simulink model "SecRwLtStLgrstInwdOtwdCtrl"  (R2018b)
settings: Solver=FixedStepDiscrete  StartTime=0.0  StopTime=10.0  FixedStep=0.01  RelTol=1e-3
undefined symbols (not defined in the file or in its folder): KeSMSuMdMotFinshdTm_Val, KeSMSuMdRetryTm1_Val, KeSMSuModeReqDurgTm_Val, KeSMSwSecRwLtStLgrstInwdOtwdEnTrigBitMask_Val
libraries: StCtrlLibBkRecln x1
settings Model: Creator=sn2xws  LastModifiedBy=sn55gm
settings Model: ModifiedHistory=|
  | 2024.10.14 V3.0.0 BitMask接口改为变量接口
  | 25.7.7 V3.13.0 Md61 Md62新增Retry口
  | 25.12.04 V3.14.0 MD10防夹后退出
settings DataIOCC: SaveFormat=StructureWithTime
settings OptimizationCC: DefaultParameterBehavior=Inlined  EnhancedBackFolding=on  PassReuseOutputArgsAs=Individual arguments  ZeroExternalMemoryAtStartup=off  ZeroInternalMemoryAtStartup=off  OptimizeBlockOrder=speed  DifferentSizesBufferReuse=on  OptimizationCustomize=off
settings DebuggingCC: ParameterTunabilityLossMsg=error
settings ModelReferenceCC: ModelReferenceNumInstancesAllowed=Single
settings SFSimCC: MATLABDynamicMemAlloc=off
settings RTWCC: SystemTargetFile=autosar.tlc  GenCodeOnly=on  TemplateMakefile=ert_default_tmf  Description=AUTOSAR  GenerateReport=on  IncludeHyperlinkInReport=on  LaunchReport=on  GenerateTraceInfo=on  GenerateTraceReport=on  GenerateTraceReportSl=on  GenerateTraceReportSf=on  GenerateTraceReportEml=on
settings CodeAppCC: ForceParamTrailComments=on  IgnoreCustomStorageClasses=off  OperatorAnnotations=on  SimulinkDataObjDesc=on  SFDataObjDesc=on  InsertBlockDesc=on
settings STFCustomTargetCC: TargetLangStandard=C99 (ISO)  MultiwordLength=256  ParMdlRefBuildCompliant=on  CompOptLevelCompliant=on  IncludeMdlTerminateFcn=off  CombineOutputUpdateFcns=on  SuppressErrorStatus=on  ERTCustomFileBanners=on  SupportNonFinite=off  SupportComplex=off  SupportContinuousTime=off  SupportNonInlinedSFcns=off  RemoveResetFunc=on  MATLABClassNameForMDSCustomization=Simulink.SoftwareTarget.ERTCustomization  AutosarCompliant=on  UseToolchainInfoCompliant=on  LookupTableObjectStructAxisOrder=2,1,3,4,...  LUTObjectStructOrderEvenSpacing=Size,Table,Breakpoints  SystemTargetFile=autosar.tlc
settings ERTTargetCC: TargetLangStandard=C99 (ISO)  ConcurrentExecutionCompliant=off  IncludeMdlTerminateFcn=off  SuppressErrorStatus=on  SupportNonFinite=off  SupportComplex=off  ModelStepFunctionPrototypeControlCompliant=off  CPPClassGenCompliant=off  AutosarCompliant=on  LookupTableObjectStructAxisOrder=2,1,3,4,...  LUTObjectStructOrderEvenSpacing=Size,Table,Breakpoints  InlinedParameterPlacement=NonHierarchical  ERTCustomFileTemplate=example_file_process.tlc  ERTFilePackagingFormat=Compact

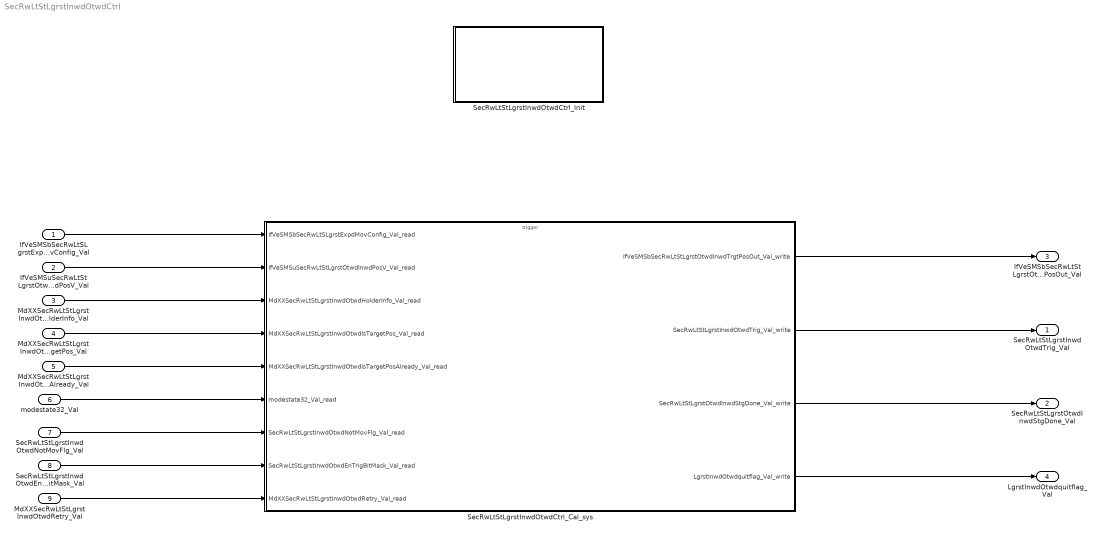
== system SecRwLtStLgrstInwdOtwdCtrl ==
  IfVeSMSbSecRwLtSLgrstExpdMovConfig_Val : Inport  OutDataTypeStr=boolean  PortDimensions=1
  IfVeSMSuSecRwLtStLgrstOtwdInwdPosV_Val : Inport  Port=2  OutDataTypeStr=boolean  PortDimensions=1
  MdXXSecRwLtStLgrstInwdOtwdHolderInfo_Val : Inport  Port=3  OutDataTypeStr=uint32  PortDimensions=1
  MdXXSecRwLtStLgrstInwdOtwdIsTargetPos_Val : Inport  Port=4  OutDataTypeStr=uint32  PortDimensions=1
  MdXXSecRwLtStLgrstInwdOtwdIsTargetPosAlready_Val : Inport  Port=5  OutDataTypeStr=uint32  PortDimensions=1
  modestate32_Val : Inport  Port=6  OutDataTypeStr=uint32  PortDimensions=1
  SecRwLtStLgrstInwdOtwdNotMovFlg_Val : Inport  Port=7  OutDataTypeStr=boolean  PortDimensions=1
  SecRwLtStLgrstInwdOtwdEnTrigBitMask_Val : Inport  Port=8  OutDataTypeStr=uint32  PortDimensions=1
  MdXXSecRwLtStLgrstInwdOtwdRetry_Val : Inport  Port=9  OutDataTypeStr=uint32  PortDimensions=1
  SecRwLtStLgrstInwdOtwdCtrl_Cal_sys : Subsystem
  SecRwLtStLgrstInwdOtwdCtrl_Init : Subsystem
  SecRwLtStLgrstInwdOtwdTrig_Val : Outport  OutDataTypeStr=boolean  PortDimensions=1
  SecRwLtStLgrstOtwdInwdStgDone_Val : Outport  Port=2  OutDataTypeStr=boolean  PortDimensions=1
  IfVeSMSbSecRwLtStLgrstOtwdInwdTrgtPosOut_Val : Outport  Port=3  OutDataTypeStr=boolean  PortDimensions=1
  LgrstInwdOtwdquitflag_Val : Outport  Port=4  OutDataTypeStr=boolean  PortDimensions=1
  wires:
  IfVeSMSbSecRwLtSLgrstExpdMovConfig_Val/1 -> SecRwLtStLgrstInwdOtwdCtrl_Cal_sys/1(IfVeSMSbSecRwLtSLgrstExpdMovConfig_Val_read)
  IfVeSMSuSecRwLtStLgrstOtwdInwdPosV_Val/1 -> SecRwLtStLgrstInwdOtwdCtrl_Cal_sys/2(IfVeSMSuSecRwLtStLgrstOtwdInwdPosV_Val_read)
  MdXXSecRwLtStLgrstInwdOtwdHolderInfo_Val/1 -> SecRwLtStLgrstInwdOtwdCtrl_Cal_sys/3(MdXXSecRwLtStLgrstInwdOtwdHolderInfo_Val_read)
  MdXXSecRwLtStLgrstInwdOtwdIsTargetPos_Val/1 -> SecRwLtStLgrstInwdOtwdCtrl_Cal_sys/4(MdXXSecRwLtStLgrstInwdOtwdIsTargetPos_Val_read)
  MdXXSecRwLtStLgrstInwdOtwdIsTargetPosAlready_Val/1 -> SecRwLtStLgrstInwdOtwdCtrl_Cal_sys/5(MdXXSecRwLtStLgrstInwdOtwdIsTargetPosAlready_Val_read)
  modestate32_Val/1 -> SecRwLtStLgrstInwdOtwdCtrl_Cal_sys/6(modestate32_Val_read)
  SecRwLtStLgrstInwdOtwdNotMovFlg_Val/1 -> SecRwLtStLgrstInwdOtwdCtrl_Cal_sys/7(SecRwLtStLgrstInwdOtwdNotMovFlg_Val_read)
  SecRwLtStLgrstInwdOtwdCtrl_Cal_sys/1(IfVeSMSbSecRwLtStLgrstOtwdInwdTrgtPosOut_Val_write) -> IfVeSMSbSecRwLtStLgrstOtwdInwdTrgtPosOut_Val/1
  SecRwLtStLgrstInwdOtwdCtrl_Cal_sys/2(SecRwLtStLgrstInwdOtwdTrig_Val_write) -> SecRwLtStLgrstInwdOtwdTrig_Val/1
  SecRwLtStLgrstInwdOtwdCtrl_Cal_sys/3(SecRwLtStLgrstOtwdInwdStgDone_Val_write) -> SecRwLtStLgrstOtwdInwdStgDone_Val/1
  SecRwLtStLgrstInwdOtwdEnTrigBitMask_Val/1 -> SecRwLtStLgrstInwdOtwdCtrl_Cal_sys/8(SecRwLtStLgrstInwdOtwdEnTrigBitMask_Val_read)
  MdXXSecRwLtStLgrstInwdOtwdRetry_Val/1 -> SecRwLtStLgrstInwdOtwdCtrl_Cal_sys/9(MdXXSecRwLtStLgrstInwdOtwdRetry_Val_read)
  SecRwLtStLgrstInwdOtwdCtrl_Cal_sys/4(LgrstInwdOtwdquitflag_Val_write) -> LgrstInwdOtwdquitflag_Val/1

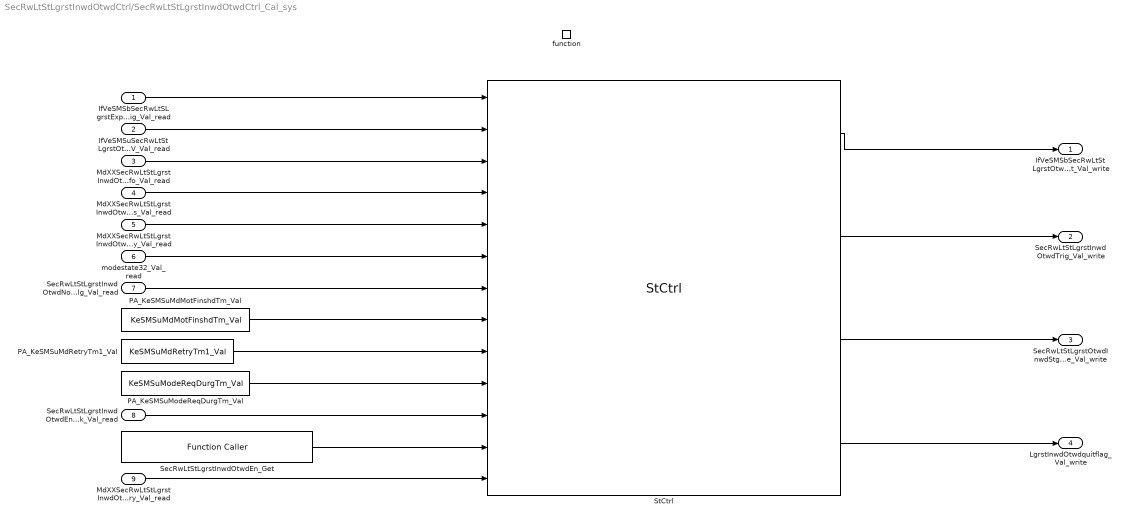
== system SecRwLtStLgrstInwdOtwdCtrl/SecRwLtStLgrstInwdOtwdCtrl_Cal_sys ==
  IfVeSMSbSecRwLtSLgrstExpdMovConfig_Val_read : Inport
  IfVeSMSuSecRwLtStLgrstOtwdInwdPosV_Val_read : Inport  Port=2
  MdXXSecRwLtStLgrstInwdOtwdHolderInfo_Val_read : Inport  Port=3
  MdXXSecRwLtStLgrstInwdOtwdIsTargetPos_Val_read : Inport  Port=4
  MdXXSecRwLtStLgrstInwdOtwdIsTargetPosAlready_Val_read : Inport  Port=5
  modestate32_Val_read : Inport  Port=6
  SecRwLtStLgrstInwdOtwdNotMovFlg_Val_read : Inport  Port=7
  SecRwLtStLgrstInwdOtwdEnTrigBitMask_Val_read : Inport  Port=8
  MdXXSecRwLtStLgrstInwdOtwdRetry_Val_read : Inport  Port=9
  function : TriggerPort  TriggerType=function-call  IsSimulinkFunction=on  FunctionName=SecRwLtStLgrstInwdOtwdCtrl_Cal  VariantControl=(inherit)
  PA_KeSMSuMdMotFinshdTm_Val : Constant  Value=KeSMSuMdMotFinshdTm_Val
  PA_KeSMSuMdRetryTm1_Val : Constant  Value=KeSMSuMdRetryTm1_Val
  PA_KeSMSuModeReqDurgTm_Val : Constant  Value=KeSMSuModeReqDurgTm_Val
  SecRwLtStLgrstInwdOtwdEn_Get : FunctionCaller  FunctionPrototype=data = SecRwLtStLgrstInwdOtwdEn_Get()  OutputArgumentSpecifications=uint32(1)
  StCtrl : StCtrlLibBkRecln/StCtrl  SystemSampleTime=-1
  IfVeSMSbSecRwLtStLgrstOtwdInwdTrgtPosOut_Val_write : Outport
      settings: EnsureOutportIsVirtual=on
  SecRwLtStLgrstInwdOtwdTrig_Val_write : Outport  Port=2
      settings: EnsureOutportIsVirtual=on
  SecRwLtStLgrstOtwdInwdStgDone_Val_write : Outport  Port=3
      settings: EnsureOutportIsVirtual=on
  LgrstInwdOtwdquitflag_Val_write : Outport  Port=4
      settings: EnsureOutportIsVirtual=on
  wires:
  StCtrl/1 -> IfVeSMSbSecRwLtStLgrstOtwdInwdTrgtPosOut_Val_write/1
  StCtrl/2 -> SecRwLtStLgrstInwdOtwdTrig_Val_write/1
  StCtrl/3 -> SecRwLtStLgrstOtwdInwdStgDone_Val_write/1
  SecRwLtStLgrstInwdOtwdEnTrigBitMask_Val_read/1 -> StCtrl/11
  SecRwLtStLgrstInwdOtwdEn_Get/1 -> StCtrl/12
  PA_KeSMSuModeReqDurgTm_Val/1 -> StCtrl/10
  PA_KeSMSuMdMotFinshdTm_Val/1 -> StCtrl/8
  PA_KeSMSuMdRetryTm1_Val/1 -> StCtrl/9
  MdXXSecRwLtStLgrstInwdOtwdIsTargetPos_Val_read/1 -> StCtrl/4
  MdXXSecRwLtStLgrstInwdOtwdIsTargetPosAlready_Val_read/1 -> StCtrl/5
  IfVeSMSbSecRwLtSLgrstExpdMovConfig_Val_read/1 -> StCtrl/1
  IfVeSMSuSecRwLtStLgrstOtwdInwdPosV_Val_read/1 -> StCtrl/2
  MdXXSecRwLtStLgrstInwdOtwdHolderInfo_Val_read/1 -> StCtrl/3
  modestate32_Val_read/1 -> StCtrl/6
  SecRwLtStLgrstInwdOtwdNotMovFlg_Val_read/1 -> StCtrl/7
  MdXXSecRwLtStLgrstInwdOtwdRetry_Val_read/1 -> StCtrl/13
  StCtrl/4 -> LgrstInwdOtwdquitflag_Val_write/1

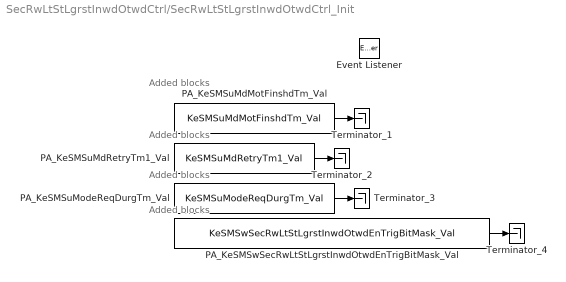
== system SecRwLtStLgrstInwdOtwdCtrl/SecRwLtStLgrstInwdOtwdCtrl_Init ==
  note: Added blocks
  note: Added blocks
  note: Added blocks
  note: Added blocks
  Event Listener : EventListener  EventName=reset
  PA_KeSMSuMdMotFinshdTm_Val : Constant  Value=KeSMSuMdMotFinshdTm_Val
  PA_KeSMSuMdRetryTm1_Val : Constant  Value=KeSMSuMdRetryTm1_Val
  PA_KeSMSuModeReqDurgTm_Val : Constant  Value=KeSMSuModeReqDurgTm_Val
  PA_KeSMSwSecRwLtStLgrstInwdOtwdEnTrigBitMask_Val : Constant  Value=KeSMSwSecRwLtStLgrstInwdOtwdEnTrigBitMask_Val
  Terminator_{1..4} (4 alike) : Terminator
  wires:
  PA_KeSMSuMdMotFinshdTm_Val/1 -> Terminator_1/1
  PA_KeSMSuMdRetryTm1_Val/1 -> Terminator_2/1
  PA_KeSMSuModeReqDurgTm_Val/1 -> Terminator_3/1
  PA_KeSMSwSecRwLtStLgrstInwdOtwdEnTrigBitMask_Val/1 -> Terminator_4/1
